simulink model "Copy_of_WK_MaoBi_Record_using_box"  (Simulink 7.7)
settings: Solver=ode4  StartTime=0.0  StopTime=inf  FixedStep=sample_time  RelTol=1e-3
InitFcn:
  | sample_time=0.005;%0.004;%0.0025;%0.02;
  | DeltaT = 0.02;
  | g = 9.81;
  | H0 = g%0.3165;
  | Kl = 1;
  | 
  | Omega_r = 1.6;%for Horizontal reference
  | Zeta_r = 0.7; %for Horizontal reference
  | Omega = 1.8;%for Horizontal Control
  | Zeta = 0.5;    %for Horizontal Control
  | 
  | Omega_h_r = 2.5; %for vertical reference
  | Zeta_h_r = 0.8;  %for vertical reference
  | Omega_h = 2.7;    %for vertical control
  | Zeta_h = 0.8;         %for vertical control
  | PI=pi;
  | 
  | Mass = 1;
  | Acc_Max = 4;
  | Acc_Max_h = 4;
  | 
  | Max_RP = 60;
undefined symbols (not defined in the file or in its folder): DiscIntNeverNeededParam
libraries: simulink x7, dspadpt3 x3, X330_Control x2, X400_Control x1
(part 2 of 2)

== stateflow chart Planning/Trajectory Logic/UAV SF ==
  state Airborne
    state TakeOff
      du:HoverThrottle = (H0 - HoverThrottle)*3*DeltaT + HoverThrottle ;
    state Initialization
      du:PosDesired[0]=InitialPos[0];PosDesired[1]=InitialPos[1];
      PosDesired[2]=InitialPos[2];
    state TrajE
      state DAQ
        en:i=0;
        du:PosShtlck[i]=Shuttlecock[0];PosShtlck[i+1]=Shuttlecock[1];
        PosShtlck[i+2]=Shuttlecock[2];PosShtlck[i+3]=Shuttlecock[3];
        PosShtlck[i+4]=Shuttlecock[4];PosShtlck[i+5]=Shuttlecock[5];i=i+6;
      state Estimation
        en:[pxe,pye,pze]=TrajEst(PosShtlck,H);
        du:PosDesired[0]=pxe;
        PosDesired[1]=pye;
        PosDesired[2]=pze;
      (default) -> DAQ
      DAQ -> Estimation : [i==30]
    state SafyHover
      en:PosDesired = Pos; PosDesired[2]=-1.2;
    state Prelanding
      en:PosDesired[0]=InitialPos[0];PosDesired[1]=InitialPos[1];
      PosDesired[2]=InitialPos[2];
    state Descent
      en:PosDesired[2] = PerchPos[2]-0.15;
    (default) -> TakeOff : {PosDesired = Pos;PosDesired[2] =-1.2;}
    TakeOff -> Initialization : after(3,sec)
    Initialization -> TrajE [order 1] : [(abs(Shuttlecock[0])<1)&(Shuttlecock[1]<2.8)&(Shuttlecock[2]<H)]
    Initialization -> SafyHover [order 2] : [RC[5] > 0]
    TrajE -> SafyHover : [(RC[5] > 0)]
    SafyHover -> Prelanding : after(3, sec)
    Prelanding -> Descent : [PerchError < 0.01]
  state Landing
    state Descending
      en:PosDesired = Pos;
      du:PosDesired[2] = (PerchPos[2]- PosDesired[2])*1*DeltaT + PosDesired[2] ;
    state CutThrottle
      du:HoverThrottle = (0 - HoverThrottle)*3*DeltaT + HoverThrottle ;
    (default) -> Descending
    Descending -> CutThrottle : [Pos[2] > (PerchPos[2]-0.1)]
  Landing -> Airborne : [RC[6] > 0.5]
  Airborne -> Landing : [RC[6] < -0.5]
  (default) -> Landing : {HoverThrottle = 0;}
  data: Shtck function_input double; xe function_output double; Hz function_input double; ye function_output double; ze function_output double; PosDesired output double size=4; HoverThrottle output double size=1; Mode output uint8 size=1; RC input double size=8; Pos input double size=4; PerchPos input double size=4; DeltaT parameter double size=1; H0 parameter double size=1; Kl parameter double size=1; VelCmd local double size=2 =0; PWM output double; PerchError input double; PI parameter double size=1; Brush input double size=3
  function [xe,ye,ze]=TrajEst(Shtck,Hz):
    | function [xe,ye,ze]=TrajEst(Shtck,Hz)
    | 
    | px=[0 0 0 0 0];
    | py=[0 0 0 0 0];
    | pz=[0 0 0 0 0];
    | vx=[0 0 0 0 0];
    | 
    | for j=1:5
    |     px(j)=Shtck(j*6-5);
    |     py(j)=Shtck(j*6-4);
    |     pz(j)=Shtck(j*6-3);
    |     vx(j)=Shtck(j*6-2);
    | end
    | 
    | x0=px(1);
    | y0=py(1);
    | sgn=sign(mean(vx));
    | dx=sgn*0.01;
    | x=-1:0.02:1;
    | y=3:-0.01:-1.5;
    | 
    | tr_zx=polyval(polyfit(px,pz,2),x);
    | tr_zy=polyval(polyfit(py,pz,2),y);
    | 
    | [~,kx]=min(abs(tr_zx-Hz));
    | [~,ky]=min(abs(tr_zy-Hz));
    | 
    | xe=x(kx);
    | ye=y(ky);
    | ze=Hz-0.1;
